simulink model "simulation_regler_lab5"  (R2020b)
settings: Solver=VariableStepAuto  StartTime=0.0  StopTime=125  RelTol=1e-3
values from neighbouring files (symbols this model uses):
  A_ans = double(subs(A,{a,b,y,f_f,f_b},{0,punkt_arb,0,ff,fb}))    [test_lab5.m]
  B_ans = double(subs(B,{a,b,y,f_f,f_b},{0,punkt_arb,0,ff,fb}))    [test_lab5.m]
  C = [1 0 0 0 0 0 ; 0 1 0 0 0 0 ;0 0 1 0 0 0]    [test_lab5.m]
  E = place(A_ans',C',p).'    [test_lab5.m]
  k_i = 1    [test_lab5.m]
  L = L.'    [test_lab5.m]
  punkt_start = deg2rad(-27)    [test_lab5.m]
undefined symbols (not defined in the file or in its folder): K_lqr
libraries: simulink_extras x9
settings Model: Creator=zhouzexu  LastModifiedBy=zhouzexu
settings DataIOCC: SaveFormat=Array  SignalLogging=off  DSMLogging=off  SaveTime=off  ReturnWorkspaceOutputs=off
settings DebuggingCC: ArithmeticOperatorsInVariantConditions=warning
settings SFSimCC: CustomCodeUndefinedFunction=UseInterfaceOnly
settings CodeAppCC: StateflowObjectComments=on

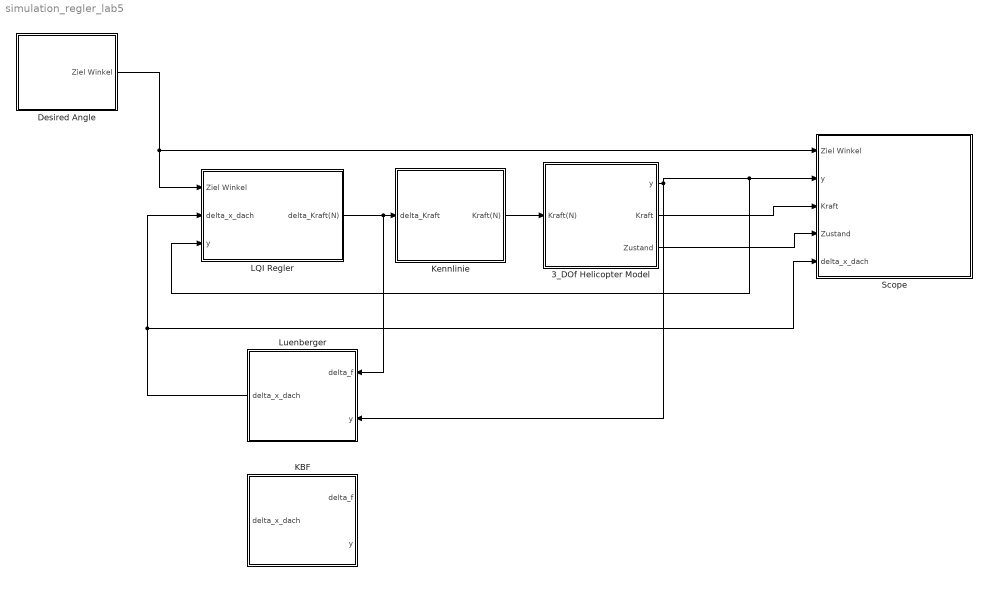
== system simulation_regler_lab5 ==
  " Kennlinie" : Subsystem
  3_DOf Helicopter Model : Subsystem
  Desired Angle : Subsystem
  "KBF " : Subsystem
  LQI Regler : Subsystem
  "Luenberger " : Subsystem
  Scope : Subsystem
  wires:
  Desired Angle/1(Ziel Winkel) -> LQI Regler/1(Ziel Winkel), Scope/1(Ziel Winkel)
  3_DOf Helicopter Model/3(Zustand) -> Scope/4(Zustand)
  3_DOf Helicopter Model/1(y) -> "Luenberger "/2(y), LQI Regler/3(y), Scope/2(y)
  3_DOf Helicopter Model/2(Kraft) -> Scope/3(Kraft)
  "Luenberger "/1(delta_x_dach) -> LQI Regler/2(delta_x_dach), Scope/5(delta_x_dach)
  LQI Regler/1(delta_Kraft(N)) -> "Luenberger "/1(delta_f), " Kennlinie"/1(delta_Kraft)
  " Kennlinie"/1(Kraft(N)) -> 3_DOf Helicopter Model/1(Kraft(N))

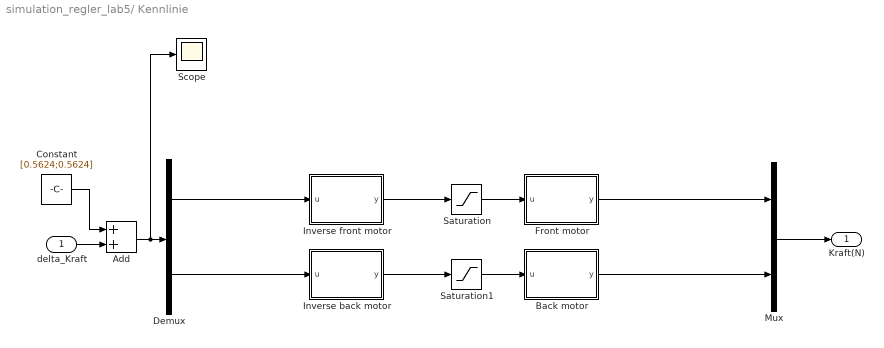
== system simulation_regler_lab5/ Kennlinie ==
  delta_Kraft : Inport
  Add : Sum
  Back motor : MATLAB Function  TreatAsAtomicUnit=on
  Constant : Constant  Value=[0.5624;0.5624]
  Demux : Demux  Outputs=2
  Front motor : MATLAB Function  TreatAsAtomicUnit=on
  Inverse back motor : MATLAB Function  TreatAsAtomicUnit=on
  Inverse front motor : MATLAB Function  TreatAsAtomicUnit=on
  Mux : Mux  Inputs=2
  Saturation : Saturate  UpperLimit=4  LowerLimit=0
  Saturation1 : Saturate  UpperLimit=4  LowerLimit=0
  Scope : Scope
  Kraft(N) : Outport
  wires:
  Mux/1 -> Kraft(N)/1
  Inverse front motor/1(y) -> Saturation/1
  Saturation/1 -> Front motor/1(u)
  Inverse back motor/1(y) -> Saturation1/1
  Saturation1/1 -> Back motor/1(u)
  Front motor/1(y) -> Mux/1
  Back motor/1(y) -> Mux/2
  Demux/2 -> Inverse back motor/1(u)
  Demux/1 -> Inverse front motor/1(u)
  Add/1 -> Scope/1, Demux/1
  delta_Kraft/1 -> Add/2
  Constant/1 -> Add/1

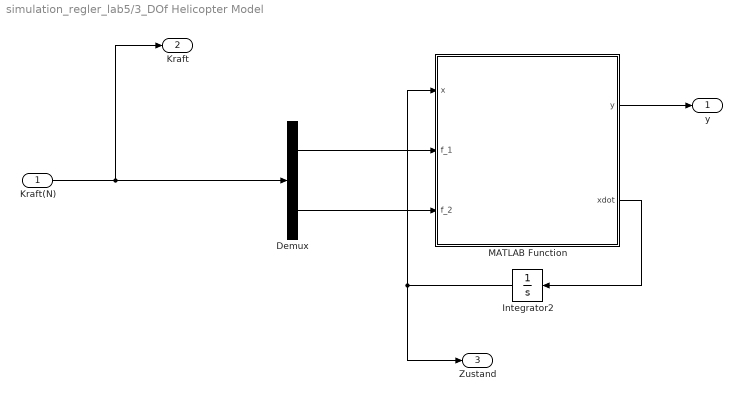
== system simulation_regler_lab5/3_DOf Helicopter Model ==
  Kraft(N) : Inport  PortDimensions=[2;1]
  Demux : Demux  Outputs=2
  Integrator2 : Integrator  InitialCondition=[0;punkt_start;0;0;0;0]
  MATLAB Function : MATLAB Function  TreatAsAtomicUnit=on
  y : Outport
  Kraft : Outport  Port=2
  Zustand : Outport  Port=3
  wires:
  Integrator2/1 -> MATLAB Function/1(x), Zustand/1
  Demux/1 -> MATLAB Function/2(f_1)
  Demux/2 -> MATLAB Function/3(f_2)
  MATLAB Function/1(y) -> y/1
  MATLAB Function/2(xdot) -> Integrator2/1
  Kraft(N)/1 -> Kraft/1, Demux/1

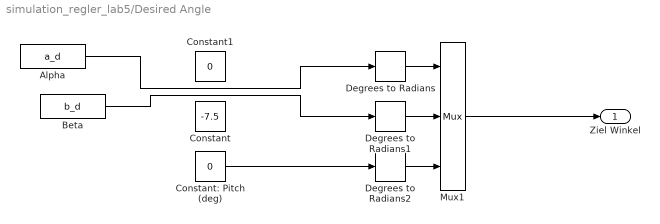
== system simulation_regler_lab5/Desired Angle ==
  Alpha : FromWorkspace  VariableName=a_d  SampleTime=0.1  OutputAfterFinalValue=Holding final value
  Beta : FromWorkspace  VariableName=b_d  SampleTime=0.1  OutputAfterFinalValue=Holding final value
  Constant : Constant  Value=-7.5
  Constant1 : Constant  Value=0
  Constant: Pitch (deg) : Constant  Value=0
  Degrees to Radians : simulink_extras/Transformations/Degrees to Radians
  Degrees to Radians1 : simulink_extras/Transformations/Degrees to Radians
  Degrees to Radians2 : simulink_extras/Transformations/Degrees to Radians
  Mux1 : Mux  Inputs=3
  Ziel Winkel : Outport
  wires:
  Mux1/1 -> Ziel Winkel/1
  Degrees to Radians/1 -> Mux1/1
  Degrees to Radians1/1 -> Mux1/2
  Degrees to Radians2/1 -> Mux1/3
  Constant: Pitch (deg)/1 -> Degrees to Radians2/1
  Alpha/1 -> Degrees to Radians/1
  Beta/1 -> Degrees to Radians1/1

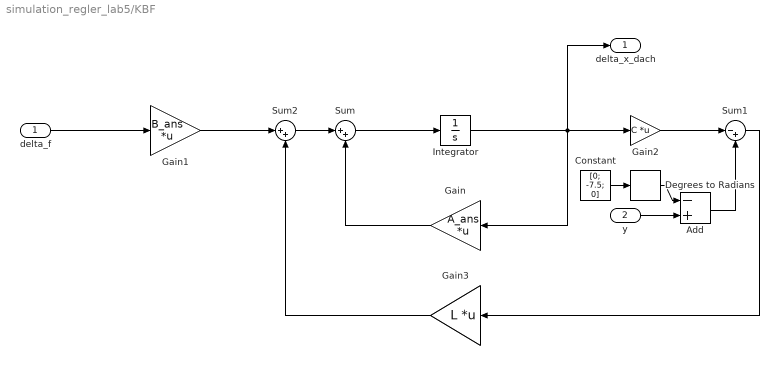
== system simulation_regler_lab5/KBF  ==
  delta_f : Inport  OutDataTypeStr=double  PortDimensions=[2;1]
  y : Inport  Port=2  PortDimensions=[3;1]
  Add : Sum  Inputs=-+
  Constant : Constant  Value=[0; -7.5; 0]
  Degrees to Radians : simulink_extras/Transformations/Degrees to Radians
  Gain : Gain  Gain=A_ans  Multiplication=Matrix(K*u)
  Gain1 : Gain  Gain=B_ans  Multiplication=Matrix(K*u)
  Gain2 : Gain  Gain=C  Multiplication=Matrix(K*u)
  Gain3 : Gain  Gain=L  Multiplication=Matrix(K*u)
  Integrator : Integrator  InitialCondition=[0;punkt_start;0;0;0;0]
  Sum : Sum  Inputs=|++
  Sum1 : Sum  Inputs=|-+
  Sum2 : Sum  Inputs=|++
  delta_x_dach : Outport  PortDimensions=[6;1]
  wires:
  Degrees to Radians/1 -> Add/1
  Constant/1 -> Degrees to Radians/1
  Add/1 -> Sum1/2
  y/1 -> Add/2
  Sum2/1 -> Sum/1
  Gain3/1 -> Sum2/2
  delta_f/1 -> Gain1/1
  Sum1/1 -> Gain3/1
  Gain2/1 -> Sum1/1
  Gain/1 -> Sum/2
  Sum/1 -> Integrator/1
  Integrator/1 -> Gain/1, Gain2/1, delta_x_dach/1
  Gain1/1 -> Sum2/1

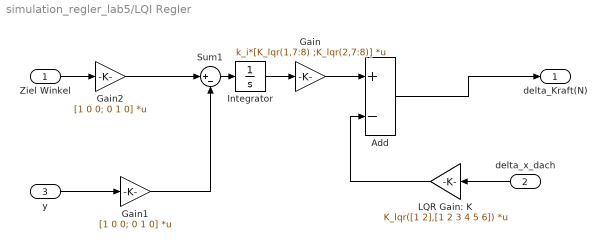
== system simulation_regler_lab5/LQI Regler ==
  Ziel Winkel : Inport
  delta_x_dach : Inport  Port=2
  y : Inport  Port=3
  Add : Sum  Inputs=+-
  Gain : Gain  Gain=k_i*[K_lqr(1,7:8) ;K_lqr(2,7:8)]  Multiplication=Matrix(K*u)
  Gain1 : Gain  Gain=[1 0 0; 0 1 0]  Multiplication=Matrix(K*u)
  Gain2 : Gain  Gain=[1 0 0; 0 1 0]  Multiplication=Matrix(K*u)
  Integrator : Integrator
  LQR Gain: K : Gain  Gain=K_lqr([1 2],[1 2 3 4 5 6])  Multiplication=Matrix(K*u)
  Sum1 : Sum  Inputs=|+-
  delta_Kraft(N) : Outport
  wires:
  delta_x_dach/1 -> LQR Gain: K/1
  LQR Gain: K/1 -> Add/2
  Add/1 -> delta_Kraft(N)/1
  Sum1/1 -> Integrator/1
  Integrator/1 -> Gain/1
  Gain1/1 -> Sum1/2
  Gain2/1 -> Sum1/1
  Ziel Winkel/1 -> Gain2/1
  y/1 -> Gain1/1
  Gain/1 -> Add/1

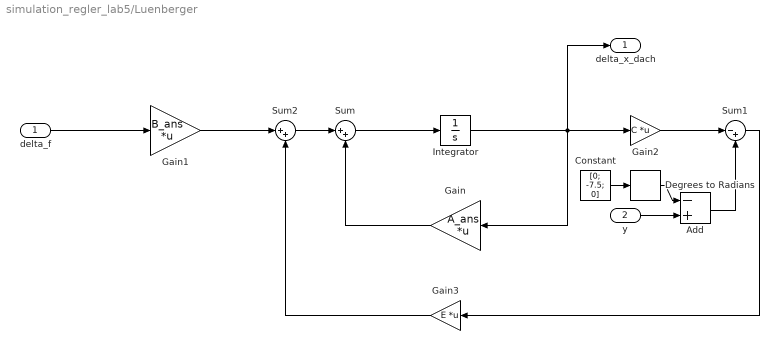
== system simulation_regler_lab5/Luenberger  ==
  delta_f : Inport  OutDataTypeStr=double  PortDimensions=[2;1]
  y : Inport  Port=2  PortDimensions=[3;1]
  Add : Sum  Inputs=-+
  Constant : Constant  Value=[0; -7.5; 0]
  Degrees to Radians : simulink_extras/Transformations/Degrees to Radians
  Gain : Gain  Gain=A_ans  Multiplication=Matrix(K*u)
  Gain1 : Gain  Gain=B_ans  Multiplication=Matrix(K*u)
  Gain2 : Gain  Gain=C  Multiplication=Matrix(K*u)
  Gain3 : Gain  Gain=E  Multiplication=Matrix(K*u)
  Integrator : Integrator  InitialCondition=[0;punkt_start;0;0;0;0]
  Sum : Sum  Inputs=|++
  Sum1 : Sum  Inputs=|-+
  Sum2 : Sum  Inputs=|++
  delta_x_dach : Outport  PortDimensions=[6;1]
  wires:
  Gain1/1 -> Sum2/1
  Integrator/1 -> delta_x_dach/1, Gain2/1, Gain/1
  Sum/1 -> Integrator/1
  Gain/1 -> Sum/2
  Gain2/1 -> Sum1/1
  Sum1/1 -> Gain3/1
  delta_f/1 -> Gain1/1
  Gain3/1 -> Sum2/2
  Sum2/1 -> Sum/1
  y/1 -> Add/2
  Add/1 -> Sum1/2
  Constant/1 -> Degrees to Radians/1
  Degrees to Radians/1 -> Add/1

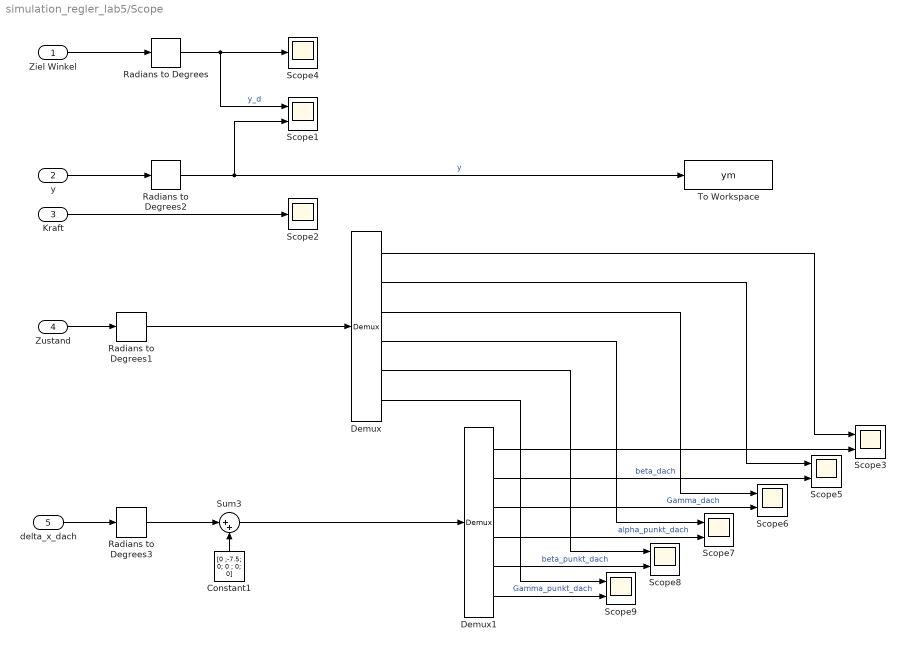
== system simulation_regler_lab5/Scope ==
  Ziel Winkel : Inport
  y : Inport  Port=2
  Kraft : Inport  Port=3
  Zustand : Inport  Port=4
  delta_x_dach : Inport  Port=5
  Constant1 : Constant  Value=[0 ;-7.5; 0; 0 ; 0; 0]
  Demux : Demux  Outputs=6
  Demux1 : Demux  Outputs=6
  Radians to Degrees{,1..3} (4 alike) : simulink_extras/Transformations/Radians to Degrees
  Scope{1,3,5..9} (7 alike) : Scope  NumInputPorts=2
  Scope2 : Scope
  Scope4 : Scope
  Sum3 : Sum  Inputs=|++
  To Workspace : ToWorkspace  VariableName=ym  SampleTime=-1
  wires:
  Kraft/1 -> Scope2/1
  Zustand/1 -> Radians to Degrees1/1
  Ziel Winkel/1 -> Radians to Degrees/1
  y/1 -> Radians to Degrees2/1
  Radians to Degrees1/1 -> Demux/1
  delta_x_dach/1 -> Radians to Degrees3/1
  Radians to Degrees2/1 -> Scope1/2, To Workspace/1  "y"
  Radians to Degrees/1 -> Scope1/1, Scope4/1  "y_d"
  Demux/1 -> Scope3/1
  Demux1/1 -> Scope3/2
  Demux/2 -> Scope5/1
  Demux1/2 -> Scope5/2  "beta_dach"
  Demux/3 -> Scope6/1
  Demux1/3 -> Scope6/2  "Gamma_dach"
  Demux/4 -> Scope7/1
  Demux1/4 -> Scope7/2  "alpha_punkt_dach"
  Demux/5 -> Scope8/1
  Demux1/5 -> Scope8/2  "beta_punkt_dach"
  Demux/6 -> Scope9/1
  Demux1/6 -> Scope9/2  "Gamma_punkt_dach"
  Radians to Degrees3/1 -> Sum3/1
  Sum3/1 -> Demux1/1
  Constant1/1 -> Sum3/2

== matlab function simulation_regler_lab5/ Kennlinie/Inverse back motor ==
  data: u input; y output
function y = fcn(u)

if u < 0
    u = 0;
end

y =sqrt(u/0.0459);

== matlab function simulation_regler_lab5/3_DOf Helicopter Model/MATLAB Function ==
  data: y output size=[3 1]; x input size=[6 1]; f_1 input size=[1 1]; xdot output size=[6 1]; f_2 input
function [y,xdot] = fcn(x,f_1,f_2)

L_g =0.042;
L_h =0.178;
L_p = 0.028;
L_a =0.655;
L_w =0.47;
L_m =0.152;
g =9.81;
M_w =1.918;
M_na = 0.240;
M_ha = 0.275;
M_m = 0.07;
M_j = 0.132;
M_h = 1.296;
M_b = 0.487;
M_f = 0.487;
M_g = 0.2;
M_motor = 0.287;
M_s = 0.322;
%% Traegheitsmoment

%gamma
% Gehaeuse
m_ge = 0.2; 
r_ge = 0.114;
h_ge = 0.027;
I_ge = 1/12* m_ge * (3*r_ge ^2 + h_ge ^2); % als ein Cylinder

%motor
m_mo = 0.287;
r_mo = 0.0195;
h_mo = 0.069;
I_mo = 1/12* m_mo * (3*r_mo ^2 + h_mo ^2); % als ein Cylinder

%schiene
m_sch = 0.322;
d_sch = 0.495;
w_sch = 0.006;
I_sch = 1/12* m_sch * (d_sch ^2 + w_sch ^2); % als ein Wuerfel

%joint
m_jo = 0.026;
d_jo = 0.019;
w_jo = 0.025;
I_jo = 1/12* m_jo * (d_jo ^2 + w_jo ^2); % als ein Wuerfel

I_y = 2*(I_ge+m_ge*((0.027/2+0.069-0.041)^2+(0.355/2)^2))+ ..., %Traegheitsmoment von Gehaeuse plus m*Distanz^2 (parallel axis theorem)
    2*(I_mo+m_mo*((0.041-0.069/2)^2+(0.355/2)^2))+ ...,%Traegheitsmoment von Motoren plus m*Distanz^2 (parallel axis theorem)
    I_sch+m_sch*(0.041+0.003)^2+ ...,%Traegheitsmoment von Schiene plus m*Distanz^2 (parallel axis theorem)
    I_jo+m_jo*(0.041-0.019/2)^2; %Traegheitsmoment von Glenke plus m*Distanz^2 (parallel axis theorem)

% elevation
L_w = 0.47; % Distance between travel axis to the counterweight
L_a = 0.655; % Distance between travel axis to the helicopter
L_g = 0.042; % Distance between elevation axis and mainarm

%gegengewicht
m_co = 1.918;
d_co = 0.070;
w_co = 0.057;
I_co = 1/12* m_co * (d_co ^2 + w_co ^2); % als Wuerfel

%hauptarm
m_ha = 0.377*(655+12.5)/915;
d_ha = L_a;
w_ha = 0.019;
I_ha = 1/12* m_ha * (d_ha ^2 + w_ha ^2);% als Wuerfel

%nebenarm
m_na = 0.377-m_ha+0.138;
d_na = L_w;
w_na = 0.019;
I_na = 1/12* m_na * (d_na ^2 + w_na ^2);% als Wuerfel

I_b = I_co + m_co * (L_w ^ 2+L_g ^2)+ ..., %Traegheitsmoment von Gegengewicht plus m*Distanz^2 (parallel axis theorem)
    I_ha + m_ha * ((L_a/2) ^ 2+L_g ^2)+ ...,%Traegheitsmoment von Hauptarm plus m*Distanz^2 (parallel axis theorem)
    I_na + m_na * ((L_w/2) ^ 2+L_g ^2)+ ...,%Traegheitsmoment von Nebenarm plus m*Distanz^2 (parallel axis theorem)
    1.322 * (L_a^2+(L_g+0.028)^2)+ ...,%Traegheitsmoment von Helicopter plus m*Distanz^2 (parallel axis theorem)
    0.07*((L_a-0.152)^2+L_g^2);%Traegheitsmoment von Magnet plus m*Distanz^2 (parallel axis theorem)

% travel 
L_h = 0.178;
m_f=0.487; %beinhalten den Gewicht vom Motor und Gehaeuse
m_b=0.487;

r = 0.114;
I_a = m_co*(L_w*cos(x(2)))^2 + 1/3*m_na*(L_w*cos(x(2)))^2+ ...,
    1/3*m_ha*(L_a*cos(x(2)))^2+1/2*(m_f+m_b)*r^2+ ...,
    (m_f+m_b)*((L_a*cos(x(2)))^2+L_h^2)+ ...,
    m_sch*(L_a*cos(x(2)))^2;
% halten Gegengewicht, Hauptarm und Nebenarm als Punkt und halten zwei
% Motoren als Cylinder
% beinhalten die Traegheitsmoment von Gegengewicht,Hauptarm, Nebenarm, Schiene und



xdot = [x(4); x(5); x(6); -(f_1+f_2)*sin(x(3))*(L_g*sin(x(2))+L_a*cos(x(2))+L_p*sin(x(2)))/I_a; ...,
    (M_w*g*cos(x(2))*L_w+M_na*g*cos(x(2))*1/2*L_w ...,
    -M_ha*g*cos(x(2))*(1/2*L_a)-M_m*g*cos(x(2))*(L_a-L_m) ...,
    -(M_h+M_j)*g*cos(x(2))*L_a-M_w*g*sin(x(2))*L_g-M_na*g*sin(x(2))*L_g ...,
    -M_ha*g*sin(x(2))*L_g-M_m*g*sin(x(2))*L_g ...,
    -(M_h+M_j)*g*sin(x(2))*(L_g+L_p)+(f_1+f_2)*cos(x(3))*L_a)/I_b; ...,
    ((f_1-f_2)*L_h+(-M_f+M_b)*g*L_h*cos(x(3))*cos(x(2)) ...,
    +M_g*2*g*cos(x(2))*sin(x(3))*(0.069+0.027/2-L_g) ...,
    -2*M_motor*g*cos(x(2))*sin(x(3))*(L_g-0.069/2)-M_s*g*cos(x(2))*sin(x(3))*L_g)/I_y];


y = [x(1); x(2);x(3)];


end

== matlab function simulation_regler_lab5/ Kennlinie/Inverse front motor ==
  data: u input; y output
function y = fcn(u)

if u<0
    u = 0;
end

y = sqrt(u/0.0599);

== matlab function simulation_regler_lab5/ Kennlinie/Front motor ==
  data: u input; y output
function y = fcn(u)

y = 0.0599*u^2;

== matlab function simulation_regler_lab5/ Kennlinie/Back motor ==
  data: u input; y output
function y = fcn(u)

y = 0.0459*u^2;
